simulink model "AI_Drivers"  (R2020b)
settings: Solver=VariableStepAuto  StartTime=0.0  StopTime=10.0  RelTol=1e-3
undefined symbols (not defined in the file): DiscIntNeverNeededParam
libraries: simulink x7, rllib x2, deeplib x1
(part 2 of 2)

== system AI_Drivers/RL Longitudinal Speed Control Type2/Signal Processing for ACC/Calculates speed error ==
  note: If the relative distance is less than the safe distance, the ego car tracks the minimum of the lead car velocity and driver-set velocity. In this manner, the ego car maintains some distance from the lead car. If the relative distance is greater than the safe distance, the ego car tracks the driver-set velocity.
  note: Lead speed
  note: e = V ref − V ego
  note: Error beween the
      | relative distance and
      | the safe distance
  note: Reference speed
  note: Ego vehicle speed
  note: Input
  note: Output
  d_err : Inport
  v_ego : Inport  Port=2
  v_lead : Inport  Port=3
  v_set : Inport  Port=4
  Min : MinMax  Inputs=2
  Scope : Scope  NumInputPorts=3
  Sum1 : Sum  Inputs=+-
  Switch : Switch  Criteria=u2 > Threshold
  v_err : Outport  VectorParamsAs1DForOutWhenUnconnected=off
  wires:
  v_ego/1 -> Sum1/2, Scope/3  "v_ego"
  Switch/1 -> Scope/2, Sum1/1  "v_ref"
  d_err/1 -> Switch/2
  v_set/1 -> Min/2, Switch/3
  Min/1 -> Switch/1
  v_lead/1 -> Min/1
  Sum1/1 -> Scope/1, v_err/1  "v_err"

== system AI_Drivers/RL Longitudinal Speed Control Type2/Signal Processing for ACC/Safe distance ==
  note: d safe =t gap ∗ V ego + D default .
  v_ego : Inport
  Default Spacing : Constant  Value=D_default  SampleTime=Ts
  Product : Product
  Sum2 : Sum
  Time Gap : Constant  Value=t_gap  SampleTime=Ts
  safe_distance : Outport  VectorParamsAs1DForOutWhenUnconnected=off
  wires:
  Sum2/1 -> safe_distance/1
  Product/1 -> Sum2/2
  Time Gap/1 -> Product/2
  Default Spacing/1 -> Sum2/1
  v_ego/1 -> Product/1

== matlab function AI_Drivers/Longitudinal Speed Control BC_LSTM/LSTM_prediction/MATLAB Function ==
  data: dataTest input; dataTest output; muFile input; sigFile input
function dataTest = fcn(dataTest, muFile, sigFile)

% Normalize the training predictors to have zero mean and unit variance
numFeatures = size(dataTest,1);

for i = 1:numFeatures
    if sigFile(i) ~= 0
        dataTest(i) = (dataTest(i) - muFile(i)) / sigFile(i);
    end
end
